simulink library "ad_blocks"  (R2017a)
settings: Solver=VariableStepAuto  StartTime=0.0  StopTime=10.0  RelTol=1e-3
undefined symbols (not defined in the file or in its folder): DiscIntNeverNeededParam
undefined symbols (not defined in the file): BatchSize, densesize, features1, features2, filtersize1
libraries: ad_blocks x23, simulink x5, dspindex x2
(part 1 of 2)
settings Model: Creator=percro2  LastModifiedBy=eruffaldi

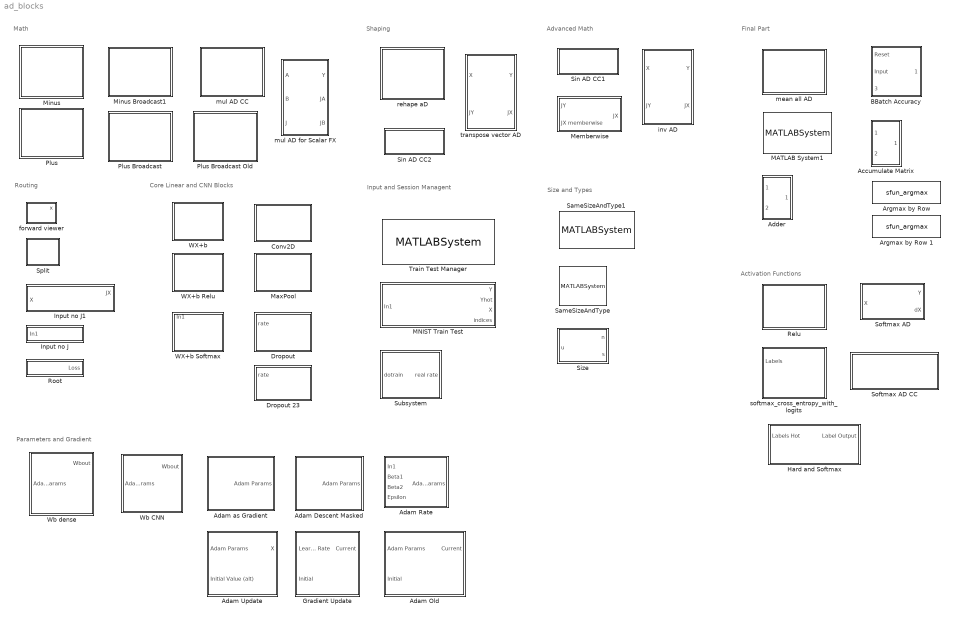
== system ad_blocks ==
  note: Advanced Math
  note: Shaping
  note: Math
  note: Size and Types
  note: Input and Session Managent
  note: Final Part
  note: Activation Functions
  note: Parameters and Gradient
  note: Routing
  note: Core Linear and CNN Blocks
  Accumulate Matrix : Subsystem  mask{Inputs=2}
      mask Callback Inputs:
      | x = gcb;
      | s = gcb;
      | asked = max(1,str2num(get_param(gcb,'Inputs')));
      | 
      | bcon = [x '/Matrix Concatenate'];
      | actual = str2num(get_param(bcon,'NumInputs'));
      | 
      | if asked == actual
      | else
      | bconL = bcon(length(x)+2:end);
      | 
      | if asked > actual
      |     set_param(bcon,'NumInputs',num2str(asked));
      |     bin1 = ([x '/In1']);
      |     bsh1 = ([x '/Reshape1']);
      |     bin1L = bin1(length(x)+2:end);
      |     bsh1L = bsh1(length(x)+2:end);
      |     for I=actual+1:asked
      |         bin = sprintf([x '/In%d'],I);
      |         bsh = sprintf([x '/Reshape%d'],I);
      |         binL = bin(length(x)+2:end);
      |         bshL = bsh(length(x)+2:end);
      |         % clone In and Reshape
      |         add_block(bin1,bin);
      |         add_block(bsh1,bsh);
      |         add_line(s,[binL '/1'],[bshL '/1']);
      |         add_line(s,[bshL '/1'],[bconL sprintf('/%d',I)]);
      |     end
      | else
      |     % remove
      |     for I=actual:-1:asked+1
      |         bin = sprintf([x '/In%d'],I);
      |         bsh = sprintf([x '/Reshape%d'],I);
      |         binL = bin(length(x)+2:end);
      |         bshL = bsh(length(x)+2:end);
      | 
      |         try
      |         delete_line(s,[binL '/1'],[bshL '/1']);
      |         catch me
      |         end
      |         try
      |         delete_line(s,[bshL '/1'],[bconL sprintf('/%d',I)]);
      |         catch me
      |         end
      |         try
      |         delete_block(bin);
      |         catch me
      |         end
      |         try
      |         delete_block(bsh);
      |         catch me
      |         end
      |     end
      |     set_param(bcon,'NumInputs',num2str(asked));
      | end
      | end
  Adam Descent Masked : Subsystem  mask{learningrate=1e-4, beta1=0.9, beta2=0.9999, epsilon=1e-8, adam=on}
      mask prompts: learningrate "Learning Rate"; adam "Check for Adam"
  Adam Old : Subsystem
  Adam Rate : Subsystem
  Adam Update : Subsystem
  Adam as Gradient : Subsystem  mask{learningrate=0.5}
  Adder : Subsystem
  "Argmax by Row " : M-S-Function  FunctionName=sfun_argmax
  Argmax by Row 1 : M-S-Function  FunctionName=sfun_argmax
  BBatch Accuracy : Subsystem
  Conv2D : Subsystem  mask{stride=[1,2,2,1], padding=-1}
      mask prompts: padding "padding (-1 auto)"
  Dropout : Subsystem
  Dropout 23 : Subsystem
  Gradient Update : Subsystem
  Hard and Softmax : Subsystem
  Input no J : Subsystem
      mask Display: disp('Input Only');
  Input no J1 : Subsystem
      mask Display: disp('Input and Gradient Only');
  MATLAB System1 : MATLABSystem  System=ArgmaxSystemD2  SimulateUsing=Code generation
      mask Type: ArgmaxSystemD2
      mask Display:
      | disp('ArgmaxSystemD2');
      | port_label('input',1,'x');
      | port_label('output',1,'y');
  MNIST Train Test : Subsystem
  MaxPool : Subsystem  mask{stride=[1,2,2,1], ksize=[1,2,2,1], padding=-1}
      mask prompts: padding "padding (-1 means auto)"
  Memberwise : Subsystem
  "Minus " : Subsystem
  Minus Broadcast1 : Subsystem
  Plus : Subsystem
  Plus Broadcast : Subsystem
  Plus Broadcast Old : Subsystem
  Relu : Subsystem
  Root : Subsystem  Description=Top level AD block: gets the incoming value, pushes the scalar 1 gradient
      mask Display: disp('Gradient Root');
  SameSizeAndType : MATLABSystem
  SameSizeAndType1 : MATLABSystem  System=samesizetype_sys  SimulateUsing=Code generation
      mask Type: samesizetype_sys
      mask Display:
      | disp('samesizetype_sys');
      | port_label('input',1,'uref');
      | port_label('input',2,'u');
      | port_label('output',1,'y');
  Sin AD CC1 : Subsystem
      mask Display: disp('inv(x)');
  Sin AD CC2 : Subsystem
      mask Display: disp('transpose(x)');
  Size : MATLAB Function  TreatAsAtomicUnit=on
  Softmax AD : Subsystem
      mask Display: image('softmax.png');
  Softmax AD CC : Subsystem
      mask Display: image('softmax.png');
  Split : Subsystem
  Subsystem : Subsystem  mask{dropout_rate=0.2}
      mask prompts: dropout_rate "Dropout Rate"
  Train Test Manager : MATLABSystem  System=train_test_mgr  testsize=10000  trainsize=60000  skiptrain=0  epochs=2  batchsize=BatchSize  SimulateUsing=Interpreted execution
      mask Type: train_test_mgr
      mask Display:
      | disp('train_test_mgr');
      | port_label('output',1,'dotrain');
      | port_label('output',2,'instop');
      | port_label('output',3,'samples');
      | port_label('output',4,'iteration');
      | port_label('output',5,'newepoch');
  "WX+b " : Subsystem
  WX+b Relu : Subsystem
  WX+b Softmax : Subsystem
  Wb CNN : Subsystem  mask{K=filtersize1, Fi=1, Fo=features1}
      mask prompts: K "Filter Size"; Fi "In Features"; Fo "Out Features"
  Wb dense : Subsystem  mask{wshape=[7*7*features2,densesize]}
      mask prompts: wshape "W Shape"
  forward viewer : Subsystem
  inv AD : Subsystem
  mean all AD : Subsystem
  mul AD CC : Subsystem
  mul AD for Scalar FX : Subsystem
  rehape aD : Subsystem  mask{shape=[-1,28,28,1]}
      mask prompts: shape "New Shape"
  softmax_cross_entropy_with_logits : Subsystem
  transpose vector AD : Subsystem

== system ad_blocks/Accumulate Matrix ==
  In1 : Inport
  In2 : Inport  Port=2
  Matrix Concatenate : Concatenate  Mode=Multidimensional array  ConcatenateDimension=2
  Reshape1 : Reshape
  Reshape2 : Reshape
  ReshapeX : Reshape  OutputDimensionality=Derive from reference input port
  Sum of Elements : Sum  Inputs=+  CollapseMode=Specified dimension  CollapseDim=2
  Out1 : Outport
  wires:
  Reshape2/1 -> Matrix Concatenate/2
  In2/1 -> Reshape2/1
  ReshapeX/1 -> Out1/1
  Matrix Concatenate/1 -> Sum of Elements/1
  Reshape1/1 -> Matrix Concatenate/1
  In1/1 -> ReshapeX/2, Reshape1/1
  Sum of Elements/1 -> ReshapeX/1

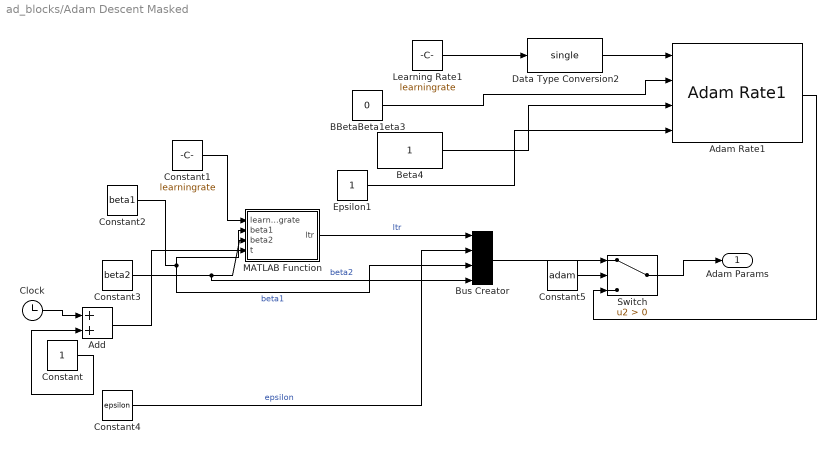
== system ad_blocks/Adam Descent Masked ==
  Adam Rate1 : ad_blocks/Adam as Gradient/Adam Rate1
  Add : Sum
  BBetaBeta1eta3 : Constant  Value=0  OutDataTypeStr=Inherit: Inherit via back propagation
  Beta4 : Constant  OutDataTypeStr=Inherit: Inherit via back propagation
  Bus Creator : BusCreator  Inputs=4
  Clock : Clock
  Constant : Constant
  Constant1 : Constant  Value=learningrate  OutDataTypeStr=Inherit: Inherit via back propagation
  Constant2 : Constant  Value=beta1  OutDataTypeStr=Inherit: Inherit via back propagation
  Constant3 : Constant  Value=beta2  OutDataTypeStr=Inherit: Inherit via back propagation
  Constant4 : Constant  Value=epsilon  OutDataTypeStr=Inherit: Inherit via back propagation
  Constant5 : Constant  Value=adam
  Data Type Conversion2 : DataTypeConversion  OutDataTypeStr=single
  Epsilon1 : Constant  OutDataTypeStr=Inherit: Inherit via back propagation
  Learning Rate1 : Constant  Value=learningrate
  MATLAB Function : MATLAB Function  TreatAsAtomicUnit=on
  Switch : Switch  Criteria=u2 > Threshold
  Adam Params : Outport
  wires:
  Constant1/1 -> MATLAB Function/1(learningrate)
  Constant2/1 -> Bus Creator/3, MATLAB Function/2(beta1)  "beta1"
  Constant3/1 -> Bus Creator/4, MATLAB Function/3(beta2)  "beta2"
  Constant4/1 -> Bus Creator/2  "epsilon"
  MATLAB Function/1(ltr) -> Bus Creator/1  "ltr"
  Constant/1 -> Add/2
  Clock/1 -> Add/1
  Add/1 -> MATLAB Function/4(t)
  Beta4/1 -> Adam Rate1/3
  BBetaBeta1eta3/1 -> Adam Rate1/2
  Epsilon1/1 -> Adam Rate1/4
  Learning Rate1/1 -> Data Type Conversion2/1
  Data Type Conversion2/1 -> Adam Rate1/1
  Bus Creator/1 -> Switch/1
  Adam Rate1/1 -> Switch/3
  Switch/1 -> Adam Params/1
  Constant5/1 -> Switch/2

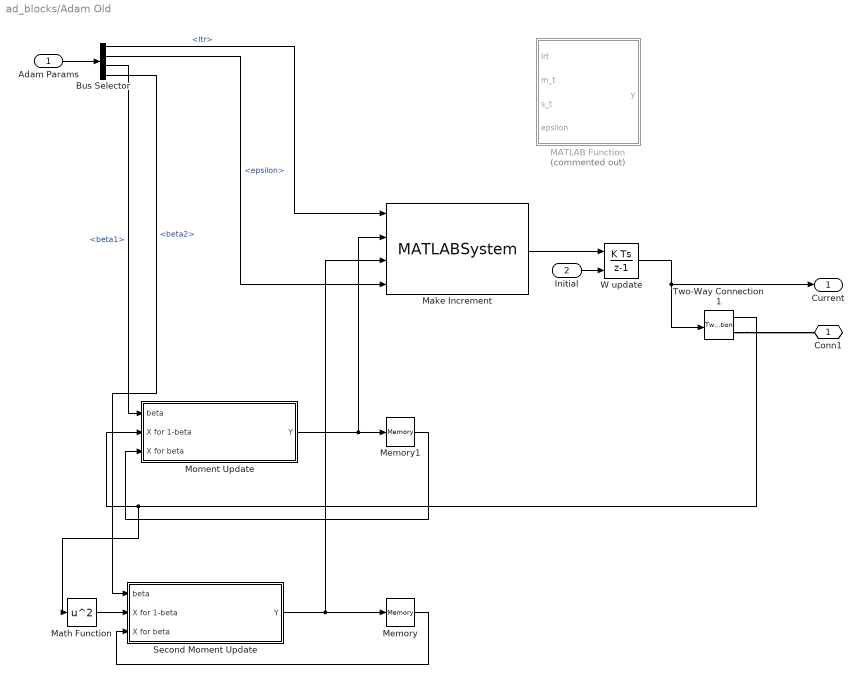
== system ad_blocks/Adam Old ==
  Adam Params : Inport
  Initial : Inport  Port=2
  Bus Selector : BusSelector  OutputSignals=ltr,epsilon,beta1,beta2
  MATLAB Function : MATLAB Function  Commented=on  TreatAsAtomicUnit=on
  Make Increment : MATLABSystem  System=adam_updateSystem  SimulateUsing=Code generation
      mask Type: adam_updateSystem
      mask Display:
      | disp('adam_updateSystem');
      | port_label('input',1,'lrt');
      | port_label('input',2,'m_t');
      | port_label('input',3,'s_t');
      | port_label('input',4,'epsilon');
      | port_label('output',1,'y');
  Math Function : Math  Operator=square  SaturateOnIntegerOverflow=on
  Memory : Memory
  Memory1 : Memory
  Moment Update : Subsystem
  Second Moment Update : Subsystem
  Two-Way Connection1 : TwoWayConnection
  W update : DiscreteIntegrator  InitialConditionSource=external  InitialConditionSetting=State (most efficient)  SampleTime=-1  ICPrevOutput=DiscIntNeverNeededParam  ICPrevScaledInput=DiscIntNeverNeededParam
  Conn1 : PMIOPort  Port=1  Side=Right
  Current : Outport
  wires:
  Make Increment/1 -> W update/1
  Bus Selector/2 -> Make Increment/4  "<epsilon>"
  Moment Update/1(Y) -> Make Increment/2, Memory1/1
  Second Moment Update/1(Y) -> Make Increment/3, Memory/1
  Math Function/1 -> Second Moment Update/2(X for 1-beta)
  Two-Way Connection1/1 -> Moment Update/2(X for 1-beta), Math Function/1
  Memory/1 -> Second Moment Update/3(X for beta)
  Bus Selector/4 -> Second Moment Update/1(beta)  "<beta2>"
  Bus Selector/3 -> Moment Update/1(beta)  "<beta1>"
  Memory1/1 -> Moment Update/3(X for beta)
  Bus Selector/1 -> Make Increment/1  "<ltr>"
  Adam Params/1 -> Bus Selector/1
  W update/1 -> Current/1, Two-Way Connection1/1
  Initial/1 -> W update/2
  connections:
  Two-Way Connection1/RConn1 -- Conn1/RConn1

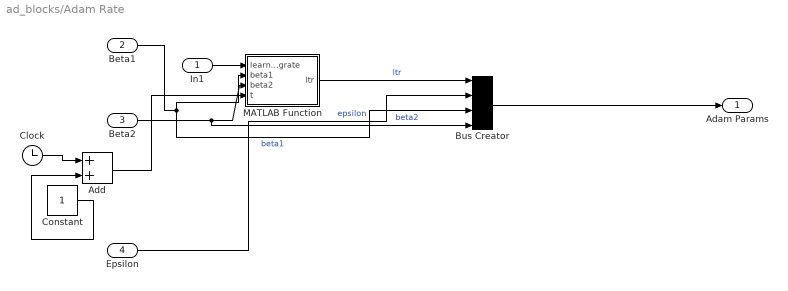
== system ad_blocks/Adam Rate ==
  In1 : Inport
  Beta1 : Inport  Port=2
  Beta2 : Inport  Port=3
  Epsilon : Inport  Port=4
  Add : Sum
  Bus Creator : BusCreator  Inputs=4
  Clock : Clock
  Constant : Constant
  MATLAB Function : MATLAB Function  TreatAsAtomicUnit=on
  Adam Params : Outport
  wires:
  In1/1 -> MATLAB Function/1(learningrate)
  Beta1/1 -> Bus Creator/3, MATLAB Function/2(beta1)  "beta1"
  Beta2/1 -> Bus Creator/4, MATLAB Function/3(beta2)  "beta2"
  Epsilon/1 -> Bus Creator/2  "epsilon"
  MATLAB Function/1(ltr) -> Bus Creator/1  "ltr"
  Bus Creator/1 -> Adam Params/1
  Constant/1 -> Add/2
  Clock/1 -> Add/1
  Add/1 -> MATLAB Function/4(t)

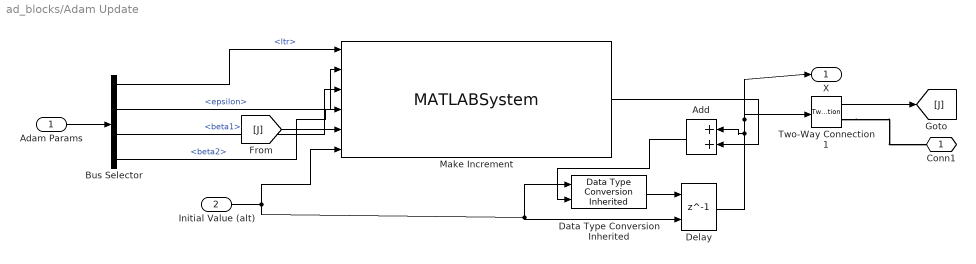
== system ad_blocks/Adam Update ==
  Adam Params : Inport
  Initial Value (alt) : Inport  Port=2
  Add : Sum  OutDataTypeStr=Inherit: Same as first input
  Bus Selector : BusSelector  OutputSignals=ltr,epsilon,beta1,beta2
  Data Type Conversion Inherited : simulink/Signal Attributes/Data Type Conversion Inherited  ConvertRealWorld=Real World Value  DoSatur=off
      settings: SourceProductName=Simulink  SourceProductBaseCode=SL
  Delay : Delay  DelayLength=1  InitialConditionSource=Input port
      settings: InputPortMap=u0,p4
  Make Increment : MATLABSystem  System=adam_updateSystem  SimulateUsing=Interpreted execution
      mask Type: adam_updateSystem
      mask Display:
      | disp('adam_updateSystem');
      | port_label('input',1,'learning_rate');
      | port_label('input',2,'epsilon');
      | port_label('input',3,'beta1');
      | port_label('input',4,'beta2');
      | port_label('input',5,'gradient');
      | port_label('input',6,'initial_for_size');
      | port_label('output',1,'effective_gradient');
  Two-Way Connection1 : TwoWayConnection
  Conn1 : PMIOPort  Port=1  Side=Right
  X : Outport
  wires:
  Adam Params/1 -> Bus Selector/1
  Bus Selector/1 -> Make Increment/1  "<ltr>"
  Bus Selector/2 -> Make Increment/2  "<epsilon>"
  Bus Selector/3 -> Make Increment/3  "<beta1>"
  Bus Selector/4 -> Make Increment/4  "<beta2>"
  Initial Value (alt)/1 -> Data Type Conversion Inherited/1, Delay/2, Make Increment/6
  Delay/1 -> Add/1, X/1, Two-Way Connection1/1
  [J] -> Make Increment/5
  Two-Way Connection1/1 -> [J]
  Make Increment/1 -> Add/2
  Data Type Conversion Inherited/1 -> Delay/1
  Add/1 -> Data Type Conversion Inherited/2
  connections:
  Two-Way Connection1/RConn1 -- Conn1/RConn1

== system ad_blocks/Adam as Gradient ==
  Adam Rate1 : Subsystem
  BBetaBeta1eta3 : Constant  Value=0  OutDataTypeStr=Inherit: Inherit via back propagation
  Beta4 : Constant  OutDataTypeStr=Inherit: Inherit via back propagation
  Data Type Conversion2 : DataTypeConversion  OutDataTypeStr=single
  Epsilon1 : Constant  OutDataTypeStr=Inherit: Inherit via back propagation
  Learning Rate1 : Constant  Value=learningrate
  Adam Params : Outport
  wires:
  Data Type Conversion2/1 -> Adam Rate1/1(In1)
  Adam Rate1/1(Adam Params) -> Adam Params/1
  Epsilon1/1 -> Adam Rate1/4(Epsilon)
  BBetaBeta1eta3/1 -> Adam Rate1/2(Beta1)
  Beta4/1 -> Adam Rate1/3(Beta2)
  Learning Rate1/1 -> Data Type Conversion2/1

== system ad_blocks/Adder ==
  Initial : Inport
  Input : Inport  Port=2
  Add : Sum
  Delay : Delay  DelayLength=1  InitialConditionSource=Input port
      settings: InputPortMap=u0,p4
  Output : Outport
  wires:
  Delay/1 -> Add/1
  Add/1 -> Output/1, Delay/1
  Initial/1 -> Delay/2
  Input/1 -> Add/2

== system ad_blocks/BBatch Accuracy ==
  Reset : Inport
  Input : Inport  Port=2
  Total Count : Inport  Port=3
  Data Type Conversion1 : DataTypeConversion
  Divide : Product  Inputs=*/
  Sum of Elements : Sum  Inputs=+
  W update : DiscreteIntegrator  ExternalReset=rising  InitialConditionSetting=State (most efficient)  SampleTime=-1  ICPrevOutput=DiscIntNeverNeededParam  ICPrevScaledInput=DiscIntNeverNeededParam
  Accuracy : Outport
  wires:
  Input/1 -> Sum of Elements/1
  W update/1 -> Divide/1
  Total Count/1 -> Divide/2
  Divide/1 -> Accuracy/1
  Sum of Elements/1 -> Data Type Conversion1/1
  Data Type Conversion1/1 -> W update/1
  Reset/1 -> W update/2

== system ad_blocks/Conv2D ==
  Gradient : MATLABSystem  System=conv2d_grad  SimulateUsing=Interpreted execution
      mask Type: conv2d_grad
      mask Display:
      | disp('conv2d_grad');
      | port_label('input',1,'U_B_Ph_Pw_Q');
      | port_label('input',2,'A_B_I_C');
      | port_label('input',3,'W_K_C_Q');
      | port_label('input',4,'Sel_PKC_IC');
      | port_label('input',5,'Xp_BP_KC');
      | port_label('output',1,'dzdx_B_Ph_Pw_Q');
      | port_label('output',2,'dzdW_K_C_Q');
  Setup : MATLABSystem  System=conv2d_setup  padding=padding  stride=stride  SimulateUsing=Interpreted execution
      mask Type: conv2d_setup
      mask Display:
      | disp('conv2d_setup');
      | port_label('input',1,'X');
      | port_label('input',2,'W');
      | port_label('output',1,'Sel_PKC_IC');
      | port_label('output',2,'Zero_Ph_Pw');
  Two-Way Connection1 : TwoWayConnection
  Two-Way Connection2 : TwoWayConnection
  Two-Way Connection3 : TwoWayConnection
  Value : MATLABSystem  System=conv2d_eval  padding=-1  stride=stride  SimulateUsing=Interpreted execution
      mask Type: conv2d_eval
      mask Display:
      | disp('conv2d_eval');
      | port_label('input',1,'A_B_I_C');
      | port_label('input',2,'W_K_C_Q');
      | port_label('input',3,'Sel_PKC_IC');
      | port_label('input',4,'Zero_Ph_PW');
      | port_label('output',1,'y_B_Ph_Pw_Q');
      | port_label('output',2,'Xp_BP_KC');
  X : PMIOPort  Port=1  Side=Left
  W : PMIOPort  Port=2  Side=Left
  Y : PMIOPort  Port=3  Side=Right
  wires:
  Two-Way Connection1/1 -> Gradient/2, Value/1, Setup/1
  Value/1 -> Two-Way Connection2/1
  Two-Way Connection3/1 -> Gradient/3, Value/2, Setup/2
  Gradient/1 -> Two-Way Connection1/1
  Gradient/2 -> Two-Way Connection3/1
  Two-Way Connection2/1 -> Gradient/1
  Value/2 -> Gradient/5
  Setup/1 -> Gradient/4, Value/3
  Setup/2 -> Value/4
  connections:
  X/RConn1 -- Two-Way Connection1/RConn1
  Two-Way Connection2/RConn1 -- Y/RConn1
  W/RConn1 -- Two-Way Connection3/RConn1

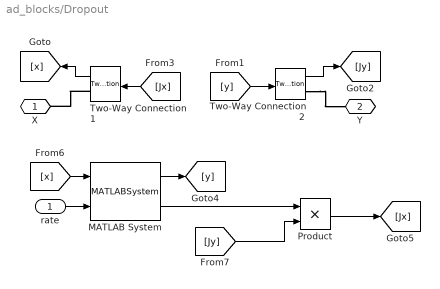
== system ad_blocks/Dropout ==
  rate : Inport
  MATLAB System : MATLABSystem  System=dropout_sys  SimulateUsing=Code generation
      mask Type: dropout_sys
      mask Display:
      | disp('dropout_sys');
      | port_label('input',1,'x');
      | port_label('input',2,'rate');
      | port_label('output',1,'y');
      | port_label('output',2,'mask');
  Product : Product
  Two-Way Connection1 : TwoWayConnection
  Two-Way Connection2 : TwoWayConnection
  X : PMIOPort  Port=1  Side=Left
  Y : PMIOPort  Port=2  Side=Right
  wires:
  rate/1 -> MATLAB System/2
  [Jx] -> Two-Way Connection1/1
  [y] -> Two-Way Connection2/1
  Two-Way Connection2/1 -> [Jy]
  Two-Way Connection1/1 -> [x]
  [x] -> MATLAB System/1
  MATLAB System/1 -> [y]
  Product/1 -> [Jx]
  MATLAB System/2 -> Product/1
  [Jy] -> Product/2
  connections:
  Two-Way Connection2/RConn1 -- Y/RConn1
  Two-Way Connection1/RConn1 -- X/RConn1

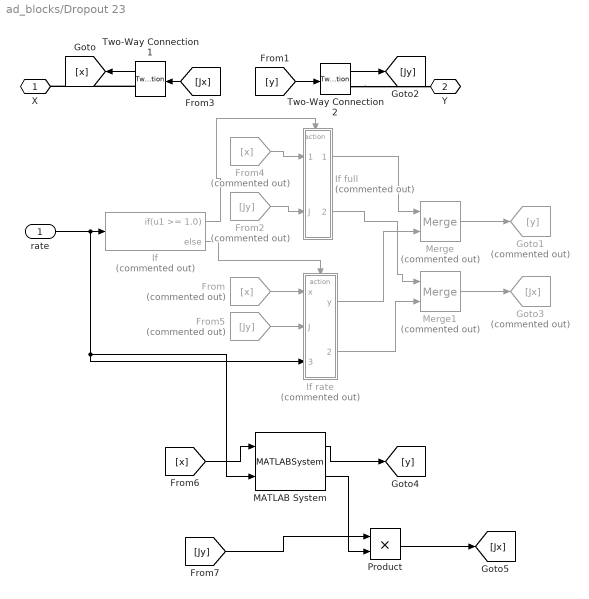
== system ad_blocks/Dropout 23 ==
  rate : Inport
  From : From  Commented=on  GotoTag=x
  From2 : From  Commented=on  GotoTag=Jy
  From4 : From  Commented=on  GotoTag=x
  From5 : From  Commented=on  GotoTag=Jy
  Goto1 : Goto  Commented=on  GotoTag=y
  Goto3 : Goto  Commented=on  GotoTag=Jx
  If : If  Commented=on  IfExpression=u1 >= 1.0
  If full : Subsystem  Commented=on  TreatAsAtomicUnit=on
  If rate : Subsystem  Commented=on  TreatAsAtomicUnit=on
  MATLAB System : MATLABSystem  System=dropout23_sys  SimulateUsing=Code generation
      mask Type: dropout23_sys
      mask Display:
      | disp('dropout23_sys');
      | port_label('input',1,'x');
      | port_label('input',2,'rate');
      | port_label('output',1,'y');
      | port_label('output',2,'mask');
  Merge : Merge  Commented=on
  Merge1 : Merge  Commented=on
  Product : Product
  Two-Way Connection1 : TwoWayConnection
  Two-Way Connection2 : TwoWayConnection
  X : PMIOPort  Port=1  Side=Left
  Y : PMIOPort  Port=2  Side=Right
  wires:
  rate/1 -> MATLAB System/2, If rate/3(rate), If/1
  If/1 -> If full/Action
  If/2 -> If rate/Action
  If full/1(y) -> Merge/1
  If rate/1(y) -> Merge/2
  If full/2(Jx) -> Merge1/1
  If rate/2(Jx) -> Merge1/2
  Merge/1 -> Goto1/1
  Merge1/1 -> Goto3/1
  [Jx] -> Two-Way Connection1/1
  [y] -> Two-Way Connection2/1
  Two-Way Connection2/1 -> [Jy]
  Two-Way Connection1/1 -> [x]
  From/1 -> If rate/1(x)
  From2/1 -> If full/2(J)
  From4/1 -> If full/1(x)
  From5/1 -> If rate/2(J)
  [x] -> MATLAB System/1
  MATLAB System/1 -> [y]
  Product/1 -> [Jx]
  MATLAB System/2 -> Product/2
  [Jy] -> Product/1
  connections:
  Two-Way Connection2/RConn1 -- Y/RConn1
  Two-Way Connection1/RConn1 -- X/RConn1

== system ad_blocks/Gradient Update ==
  Learning Rate : Inport
  Initial : Inport  Port=2
  Adder : ad_blocks/Adder
  Product : Product
  Two-Way Connection1 : TwoWayConnection
  Unary Minus : UnaryMinus
  Conn1 : PMIOPort  Port=1  Side=Right
  Current : Outport
  wires:
  Learning Rate/1 -> Unary Minus/1
  Two-Way Connection1/1 -> Product/1
  Adder/1 -> Current/1, Two-Way Connection1/1
  Unary Minus/1 -> Product/2
  Initial/1 -> Adder/1
  Product/1 -> Adder/2
  connections:
  Two-Way Connection1/RConn1 -- Conn1/RConn1

== system ad_blocks/Hard and Softmax ==
  Labels Hot : Inport
  MATLAB System1 : ad_blocks/MATLAB System1  SimulateUsing=Code generation
  forward viewer2 : ad_blocks/forward viewer  SystemSampleTime=-1
  softmax_cross_entropy_with_logits : ad_blocks/softmax_cross_entropy_with_logits
  X : PMIOPort  Port=1  Side=Left
  Y : PMIOPort  Port=2  Side=Right
  Label Output : Outport
  wires:
  forward viewer2/1 -> MATLAB System1/1
  Labels Hot/1 -> softmax_cross_entropy_with_logits/1
  MATLAB System1/1 -> Label Output/1
  connections:
  softmax_cross_entropy_with_logits/RConn1 -- Y/RConn1
  forward viewer2/RConn1 -- softmax_cross_entropy_with_logits/LConn1
  X/RConn1 -- forward viewer2/LConn1

== system ad_blocks/Input no J ==
  In1 : Inport
  Terminator : Terminator
  Two-Way Connection1 : TwoWayConnection
  Conn1 : PMIOPort  Port=1  Side=Right
  wires:
  In1/1 -> Two-Way Connection1/1
  Two-Way Connection1/1 -> Terminator/1
  connections:
  Conn1/RConn1 -- Two-Way Connection1/RConn1

== system ad_blocks/Input no J1 ==
  X : Inport
  Two-Way Connection1 : TwoWayConnection
  (X,JX) : PMIOPort  Port=1  Side=Right
  JX : Outport
  wires:
  Two-Way Connection1/1 -> JX/1
  X/1 -> Two-Way Connection1/1
  connections:
  (X,JX)/RConn1 -- Two-Way Connection1/RConn1

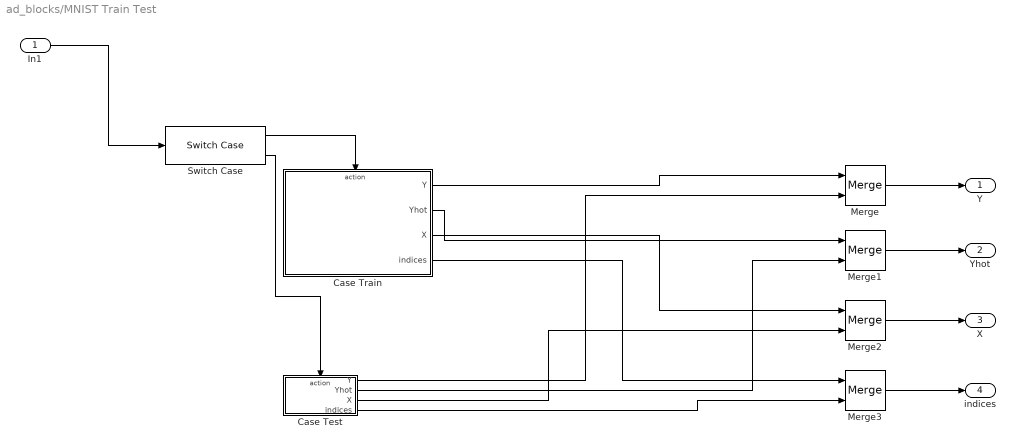
== system ad_blocks/MNIST Train Test ==
  In1 : Inport
  Case Test : Subsystem  TreatAsAtomicUnit=on
  Case Train : Subsystem  TreatAsAtomicUnit=on
  Merge{,1..3} (4 alike) : Merge
  Switch Case : SwitchCase
  "Y " : Outport
  Yhot : Outport  Port=2
  X : Outport  Port=3
  indices : Outport  Port=4
  wires:
  In1/1 -> Switch Case/1
  Switch Case/1 -> Case Train/Action
  Switch Case/2 -> Case Test/Action
  Case Train/1(Y) -> Merge/1
  Case Train/2(Yhot) -> Merge1/1
  Case Train/3(X) -> Merge2/1
  Case Test/1(Y) -> Merge/2
  Case Test/2(Yhot) -> Merge1/2
  Case Test/3(X) -> Merge2/2
  Merge/1 -> "Y "/1
  Merge1/1 -> Yhot/1
  Merge2/1 -> X/1
  Merge3/1 -> indices/1
  Case Test/4(indices) -> Merge3/2
  Case Train/4(indices) -> Merge3/1

== system ad_blocks/MaxPool ==
  note: setup is based on the constant size extraction, then it produces in a constant way the indices
      | then the evaluation produces also the indices I that are finally used in the gradient
  Gradient : MATLABSystem  System=maxpool_grad  ksize=ksize  strides=stride  SimulateUsing=Interpreted execution
      mask Type: maxpool_grad
      mask Display:
      | disp('maxpool_grad');
      | port_label('input',1,'U_B_Ph_Pw_Q');
      | port_label('input',2,'argmaxbase');
      | port_label('input',3,'maxindices_BPC');
      | port_label('input',4,'argmaxbasescale');
      | port_label('input',5,'Zero_Ph_Pw');
      | port_label('input',6,'X_B_I_C');
      | port_label('input',7,'Sel_PCK_IC');
      | port_label('input',8,'Sel_PCK_IC_A');
      | port_label('output',1,'J_BIC');
  Setup : MATLABSystem  System=maxpool_setup  ksize=ksize  strides=stride  padding=padding  SimulateUsing=Interpreted execution
      mask Type: maxpool_setup
      mask Display:
      | disp('maxpool_setup');
      | port_label('input',1,'X');
      | port_label('output',1,'Sel_PCK_IC');
      | port_label('output',2,'argmaxbase');
      | port_label('output',3,'argmaxbasescale');
      | port_label('output',4,'Zero_Ph_Pw');
      | port_label('output',5,'Sel_PCK_IC_A');
  Two-Way Connection1 : TwoWayConnection
  Two-Way Connection2 : TwoWayConnection
  "Value " : MATLABSystem  System=maxpool_eval  strides=stride  ksize=ksize  SimulateUsing=Interpreted execution
      mask Type: maxpool_eval
      mask Display:
      | disp('maxpool_eval');
      | port_label('input',1,'X_B_I_C');
      | port_label('input',2,'Sel_PCK_IC');
      | port_label('input',3,'Zero_Ph_Pw');
      | port_label('output',1,'y_B_P_C');
      | port_label('output',2,'maxindices_BPC');
  X : PMIOPort  Port=1  Side=Left
  Y : PMIOPort  Port=2  Side=Right
  wires:
  Two-Way Connection1/1 -> Setup/1, Gradient/6, "Value "/1
  Gradient/1 -> Two-Way Connection1/1
  "Value "/1 -> Two-Way Connection2/1
  Setup/1 -> Gradient/7, "Value "/2
  Two-Way Connection2/1 -> Gradient/1
  Setup/2 -> Gradient/2
  Setup/4 -> "Value "/3, Gradient/5
  Setup/3 -> Gradient/4
  "Value "/2 -> Gradient/3
  Setup/5 -> Gradient/8
  connections:
  Y/RConn1 -- Two-Way Connection2/RConn1
  X/RConn1 -- Two-Way Connection1/RConn1

== system ad_blocks/Memberwise ==
  JY : Inport
  JX memberwise : Inport  Port=2
  Product : Product
  JX : Outport
  wires:
  JY/1 -> Product/1
  JX memberwise/1 -> Product/2
  Product/1 -> JX/1

== system ad_blocks/Minus  ==
  Add : Sum  Inputs=+-
  Gain : Gain  Gain=-1
  Two-Way Connection1 : TwoWayConnection
  Two-Way Connection2 : TwoWayConnection
  Two-Way Connection4 : TwoWayConnection
  A : PMIOPort  Port=1  Side=Left
  B : PMIOPort  Port=2  Side=Left
  Y : PMIOPort  Port=3  Side=Right
  wires:
  Two-Way Connection2/1 -> Add/1
  Two-Way Connection1/1 -> Gain/1, Two-Way Connection2/1
  Add/1 -> Two-Way Connection1/1
  Gain/1 -> Two-Way Connection4/1
  Two-Way Connection4/1 -> Add/2
  connections:
  Y/RConn1 -- Two-Way Connection1/RConn1
  Two-Way Connection4/RConn1 -- B/RConn1
  A/RConn1 -- Two-Way Connection2/RConn1

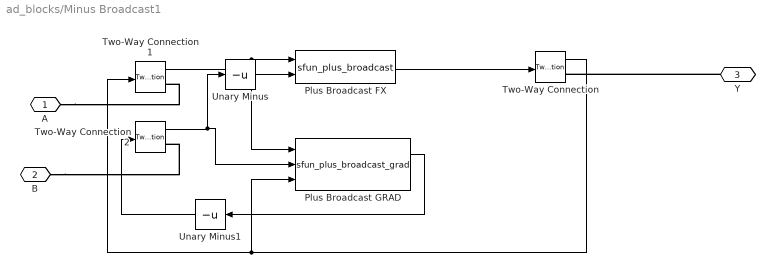
== system ad_blocks/Minus Broadcast1 ==
  Plus Broadcast FX : M-S-Function  FunctionName=sfun_plus_broadcast
  Plus Broadcast GRAD : M-S-Function  FunctionName=sfun_plus_broadcast_grad
  Two-Way Connection : TwoWayConnection
  Two-Way Connection1 : TwoWayConnection
  Two-Way Connection2 : TwoWayConnection
  Unary Minus : UnaryMinus
  Unary Minus1 : UnaryMinus
  A : PMIOPort  Port=1  Side=Left
  B : PMIOPort  Port=2  Side=Left
  Y : PMIOPort  Port=3  Side=Right
  wires:
  Two-Way Connection/1 -> Plus Broadcast GRAD/3, Two-Way Connection1/1
  Plus Broadcast GRAD/1 -> Unary Minus1/1
  Two-Way Connection2/1 -> Unary Minus/1, Plus Broadcast GRAD/2
  Two-Way Connection1/1 -> Plus Broadcast FX/1, Plus Broadcast GRAD/1
  Plus Broadcast FX/1 -> Two-Way Connection/1
  Unary Minus/1 -> Plus Broadcast FX/2
  Unary Minus1/1 -> Two-Way Connection2/1
  connections:
  B/RConn1 -- Two-Way Connection2/RConn1
  A/RConn1 -- Two-Way Connection1/RConn1
  Y/RConn1 -- Two-Way Connection/RConn1

== system ad_blocks/Plus ==
  Add : Sum
  Two-Way Connection : TwoWayConnection
  Two-Way Connection1 : TwoWayConnection
  Two-Way Connection2 : TwoWayConnection
  A : PMIOPort  Port=1  Side=Left
  B : PMIOPort  Port=2  Side=Left
  Y : PMIOPort  Port=3  Side=Right
  wires:
  Two-Way Connection2/1 -> Add/2
  Two-Way Connection1/1 -> Add/1
  Two-Way Connection/1 -> Two-Way Connection2/1, Two-Way Connection1/1
  Add/1 -> Two-Way Connection/1
  connections:
  B/RConn1 -- Two-Way Connection2/RConn1
  A/RConn1 -- Two-Way Connection1/RConn1
  Y/RConn1 -- Two-Way Connection/RConn1

== system ad_blocks/Plus Broadcast ==
  Two-Way Connection : TwoWayConnection
  Two-Way Connection1 : TwoWayConnection
  Two-Way Connection2 : TwoWayConnection
  function : MATLABSystem  System=SumBroadcast  SimulateUsing=Code generation
      mask Type: SumBroadcast
      mask Display:
      | disp('SumBroadcast');
      | port_label('input',1,'ul');
      | port_label('input',2,'ur');
      | port_label('output',1,'y');
  gradient : MATLABSystem  System=SumBroadcastGrad  SimulateUsing=Code generation
      mask Type: SumBroadcastGrad
      mask Display:
      | disp('SumBroadcastGrad');
      | port_label('input',1,'ul');
      | port_label('input',2,'ur');
      | port_label('input',3,'J');
      | port_label('output',1,'Jl');
      | port_label('output',2,'Jr');
  A : PMIOPort  Port=1  Side=Left
  B : PMIOPort  Port=2  Side=Left
  Y : PMIOPort  Port=3  Side=Right
  wires:
  function/1 -> Two-Way Connection/1
  Two-Way Connection1/1 -> gradient/1, function/1
  Two-Way Connection2/1 -> function/2, gradient/2
  gradient/2 -> Two-Way Connection2/1
  Two-Way Connection/1 -> gradient/3
  gradient/1 -> Two-Way Connection1/1
  connections:
  Y/RConn1 -- Two-Way Connection/RConn1
  A/RConn1 -- Two-Way Connection1/RConn1
  B/RConn1 -- Two-Way Connection2/RConn1

== system ad_blocks/Plus Broadcast Old ==
  Plus Broadcast FX : M-S-Function  FunctionName=sfun_plus_broadcast
  Plus Broadcast GRAD : M-S-Function  FunctionName=sfun_plus_broadcast_grad
  Two-Way Connection : TwoWayConnection
  Two-Way Connection1 : TwoWayConnection
  Two-Way Connection2 : TwoWayConnection
  A : PMIOPort  Port=1  Side=Left
  B : PMIOPort  Port=2  Side=Left
  Y : PMIOPort  Port=3  Side=Right
  wires:
  Plus Broadcast FX/1 -> Two-Way Connection/1
  Two-Way Connection1/1 -> Plus Broadcast GRAD/1, Plus Broadcast FX/1
  Two-Way Connection2/1 -> Plus Broadcast GRAD/2, Plus Broadcast FX/2
  Plus Broadcast GRAD/1 -> Two-Way Connection2/1
  Two-Way Connection/1 -> Two-Way Connection1/1, Plus Broadcast GRAD/3
  connections:
  Y/RConn1 -- Two-Way Connection/RConn1
  A/RConn1 -- Two-Way Connection1/RConn1
  B/RConn1 -- Two-Way Connection2/RConn1

== system ad_blocks/Relu ==
  MATLAB System : MATLABSystem  System=ReluGradient_sys  SimulateUsing=Code generation
      mask Type: ReluGradient_sys
      mask Display:
      | disp('ReluGradient_sys');
      | port_label('input',1,'X');
      | port_label('input',2,'JY');
      | port_label('output',1,'JX');
  Two-Way Connection1 : TwoWayConnection
  Two-Way Connection2 : TwoWayConnection
  max(x,0) : MATLABSystem  System=Max0System  SimulateUsing=Code generation
      mask Type: Max0System
      mask Display:
      | disp('Max0System');
      | port_label('input',1,'x');
      | port_label('output',1,'y');
  X : PMIOPort  Port=1  Side=Left
  Y : PMIOPort  Port=2  Side=Right
  wires:
  Two-Way Connection1/1 -> MATLAB System/1, max(x,0)/1
  max(x,0)/1 -> Two-Way Connection2/1
  MATLAB System/1 -> Two-Way Connection1/1
  Two-Way Connection2/1 -> MATLAB System/2
  connections:
  X/RConn1 -- Two-Way Connection1/RConn1
  Two-Way Connection2/RConn1 -- Y/RConn1

== system ad_blocks/Root ==
  Constant1 : Constant  OutDataTypeStr=single
  Signal Specification : SignalSpecification  Dimensions=1
  Two-Way Connection1 : TwoWayConnection
  Conn1 : PMIOPort  Port=1  Side=Left
  Loss : Outport
  wires:
  Signal Specification/1 -> Loss/1
  Two-Way Connection1/1 -> Signal Specification/1
  Constant1/1 -> Two-Way Connection1/1
  connections:
  Conn1/RConn1 -- Two-Way Connection1/RConn1

== system ad_blocks/Sin AD CC1 ==
  Two-Way Connection : TwoWayConnection
  Two-Way Connection1 : TwoWayConnection
  inv AD : ad_blocks/inv AD
  X : PMIOPort  Port=1  Side=Left
  Y : PMIOPort  Port=2  Side=Right
  wires:
  inv AD/1 -> Two-Way Connection/1
  Two-Way Connection/1 -> inv AD/2
  Two-Way Connection1/1 -> inv AD/1
  inv AD/2 -> Two-Way Connection1/1
  connections:
  X/RConn1 -- Two-Way Connection1/RConn1
  Y/RConn1 -- Two-Way Connection/RConn1

== system ad_blocks/Sin AD CC2 ==
  Two-Way Connection : TwoWayConnection
  Two-Way Connection1 : TwoWayConnection
  transpose vector AD : ad_blocks/transpose vector AD
  X : PMIOPort  Port=1  Side=Left
  Y : PMIOPort  Port=2  Side=Right
  wires:
  transpose vector AD/2 -> Two-Way Connection1/1
  Two-Way Connection1/1 -> transpose vector AD/1
  Two-Way Connection/1 -> transpose vector AD/2
  transpose vector AD/1 -> Two-Way Connection/1
  connections:
  Y/RConn1 -- Two-Way Connection/RConn1
  X/RConn1 -- Two-Way Connection1/RConn1

== system ad_blocks/Softmax AD ==
  note: http://eli.thegreenplace.net/2016/the-softmax-function-and-its-derivative/
  note: https://github.com/Theano/Theano/blob/master/theano/tensor/nnet/nnet.py
  X : Inport
  MATLAB Function1 : MATLAB Function  TreatAsAtomicUnit=on
  MATLAB Function2 : MATLAB Function  TreatAsAtomicUnit=on
  Y : Outport
  dX : Outport  Port=2
  wires:
  MATLAB Function2/1(y) -> dX/1
  X/1 -> MATLAB Function1/1(u), MATLAB Function2/1(u)
  MATLAB Function1/1(y) -> Y/1

== system ad_blocks/Softmax AD CC ==
  Memberwise : ad_blocks/Memberwise
  Softmax AD : ad_blocks/Softmax AD  SystemSampleTime=-1
  Two-Way Connection : TwoWayConnection
  Two-Way Connection1 : TwoWayConnection
  X : PMIOPort  Port=1  Side=Left
  Y : PMIOPort  Port=2  Side=Right
  wires:
  Softmax AD/1 -> Two-Way Connection/1
  Two-Way Connection1/1 -> Softmax AD/1
  Two-Way Connection/1 -> Memberwise/1
  Memberwise/1 -> Two-Way Connection1/1
  Softmax AD/2 -> Memberwise/2
  connections:
  Y/RConn1 -- Two-Way Connection/RConn1
  X/RConn1 -- Two-Way Connection1/RConn1

== system ad_blocks/Split ==
  note: Alternatively use Clone Output
  Acciumulate Matrix : ad_blocks/Acciumulate Matrix  Inputs=2
  Two-Way Connection1 : TwoWayConnection
  Two-Way Connection2 : TwoWayConnection
  Two-Way Connection3 : TwoWayConnection
  X : PMIOPort  Port=1  Side=Left
  X1 : PMIOPort  Port=2  Side=Right
  X2 : PMIOPort  Port=3  Side=Right
  wires:
  Acciumulate Matrix/1 -> Two-Way Connection2/1
  Two-Way Connection1/1 -> Acciumulate Matrix/2
  Two-Way Connection3/1 -> Acciumulate Matrix/1
  Two-Way Connection2/1 -> Two-Way Connection3/1, Two-Way Connection1/1
  connections:
  Two-Way Connection3/RConn1 -- X2/RConn1
  X1/RConn1 -- Two-Way Connection1/RConn1
  Two-Way Connection2/RConn1 -- X/RConn1

== system ad_blocks/Subsystem ==
  dotrain : Inport
  Constant : Constant  Value=dropout_rate
  Constant1 : Constant  Value=1.0
  Switch : Switch  Criteria=u2 ~= 0
  real rate : Outport
  wires:
  Constant1/1 -> Switch/3
  Constant/1 -> Switch/1
  dotrain/1 -> Switch/2
  Switch/1 -> real rate/1

== system ad_blocks/WX+b  ==
  Plus Broadcast : ad_blocks/Plus Broadcast
  mul AD CC : ad_blocks/mul AD CC
  X : PMIOPort  Port=1  Side=Left
  W : PMIOPort  Port=2  Side=Left
  Y : PMIOPort  Port=3  Side=Right
  b : PMIOPort  Port=4  Side=Left
  connections:
  Y/RConn1 -- Plus Broadcast/RConn1
  Plus Broadcast/LConn2 -- b/RConn1
  mul AD CC/LConn1 -- X/RConn1
  mul AD CC/LConn2 -- W/RConn1
  Plus Broadcast/LConn1 -- mul AD CC/RConn1

== system ad_blocks/WX+b Relu ==
  Plus Broadcast : ad_blocks/Plus Broadcast
  Relu : ad_blocks/Relu
  mul AD CC : ad_blocks/mul AD CC
  X : PMIOPort  Port=1  Side=Left
  W : PMIOPort  Port=2  Side=Left
  Y : PMIOPort  Port=3  Side=Right
  b : PMIOPort  Port=4  Side=Left
  connections:
  Relu/RConn1 -- Y/RConn1
  Plus Broadcast/LConn2 -- b/RConn1
  mul AD CC/LConn1 -- X/RConn1
  mul AD CC/LConn2 -- W/RConn1
  Plus Broadcast/RConn1 -- Relu/LConn1
  Plus Broadcast/LConn1 -- mul AD CC/RConn1

== system ad_blocks/WX+b Softmax ==
  In1 : Inport
  Plus Broadcast : ad_blocks/Plus Broadcast
  mul AD CC : ad_blocks/mul AD CC
  softmax_cross_entropy_with_logits : ad_blocks/softmax_cross_entropy_with_logits
  X : PMIOPort  Port=1  Side=Left
  W : PMIOPort  Port=2  Side=Left
  Y : PMIOPort  Port=3  Side=Right
  b : PMIOPort  Port=4  Side=Left
  wires:
  In1/1 -> softmax_cross_entropy_with_logits/1
  connections:
  Plus Broadcast/LConn1 -- mul AD CC/RConn1
  Plus Broadcast/RConn1 -- softmax_cross_entropy_with_logits/LConn1
  mul AD CC/LConn2 -- W/RConn1
  mul AD CC/LConn1 -- X/RConn1
  Plus Broadcast/LConn2 -- b/RConn1
  softmax_cross_entropy_with_logits/RConn1 -- Y/RConn1

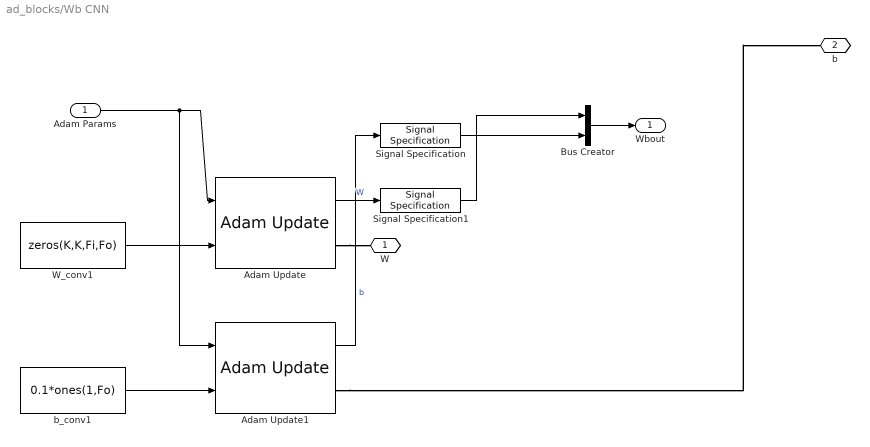
== system ad_blocks/Wb CNN ==
  Adam Params : Inport
  Adam Update : ad_blocks/Adam Update
  Adam Update1 : ad_blocks/Adam Update
  Bus Creator : BusCreator  Inputs=2
  Signal Specification : SignalSpecification  Dimensions=[Fo]
  Signal Specification1 : SignalSpecification  Dimensions=[K,K,Fi,Fo]
  W_conv1 : Constant  Value=zeros(K,K,Fi,Fo)  OutDataTypeStr=single
  b_conv1 : Constant  Value=0.1*ones(1,Fo)  OutDataTypeStr=single
  W : PMIOPort  Port=1  Side=Right
  b : PMIOPort  Port=2  Side=Right
  Wbout : Outport
  wires:
  b_conv1/1 -> Adam Update1/2
  W_conv1/1 -> Adam Update/2
  Adam Params/1 -> Adam Update/1, Adam Update1/1
  Adam Update/1 -> Signal Specification1/1  "W"
  Bus Creator/1 -> Wbout/1
  Adam Update1/1 -> Signal Specification/1  "b"
  Signal Specification/1 -> Bus Creator/2
  Signal Specification1/1 -> Bus Creator/1
  connections:
  Adam Update1/RConn1 -- b/RConn1
  Adam Update/RConn1 -- W/RConn1

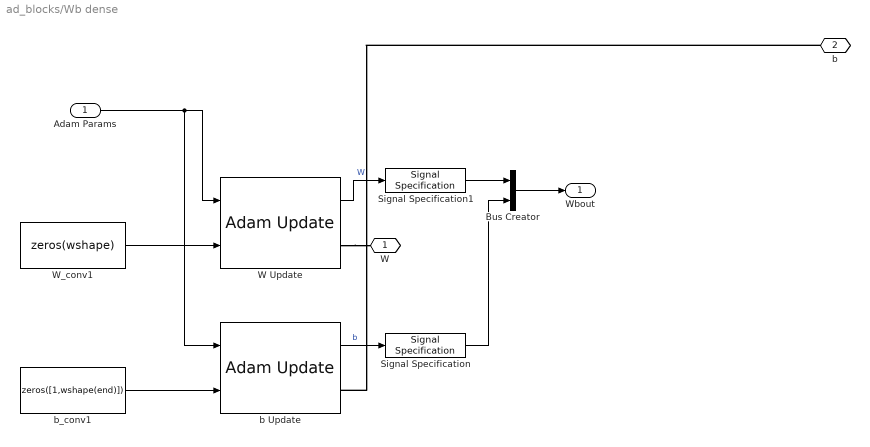
== system ad_blocks/Wb dense ==
  Adam Params : Inport
  Bus Creator : BusCreator  Inputs=2
  Signal Specification : SignalSpecification  Dimensions=[wshape(end)]
  Signal Specification1 : SignalSpecification  Dimensions=wshape
  W Update : ad_blocks/Adam Update
  W_conv1 : Constant  Value=zeros(wshape)  OutDataTypeStr=single
  b Update : ad_blocks/Adam Update
  b_conv1 : Constant  Value=zeros([1,wshape(end)])  OutDataTypeStr=single
  W : PMIOPort  Port=1  Side=Right
  b : PMIOPort  Port=2  Side=Right
  Wbout : Outport
  wires:
  b_conv1/1 -> b Update/2
  W_conv1/1 -> W Update/2
  Adam Params/1 -> b Update/1, W Update/1
  Bus Creator/1 -> Wbout/1
  W Update/1 -> Signal Specification1/1  "W"
  b Update/1 -> Signal Specification/1  "b"
  Signal Specification/1 -> Bus Creator/2
  Signal Specification1/1 -> Bus Creator/1
  connections:
  b/RConn1 -- b Update/RConn1
  W Update/RConn1 -- W/RConn1

== system ad_blocks/forward viewer ==
  Two-Way Connection1 : TwoWayConnection
  Two-Way Connection2 : TwoWayConnection
  X : PMIOPort  Port=1  Side=Left
  Y : PMIOPort  Port=2  Side=Right
  x : Outport
  wires:
  Two-Way Connection1/1 -> Two-Way Connection2/1
  Two-Way Connection2/1 -> x/1, Two-Way Connection1/1
  connections:
  Y/RConn1 -- Two-Way Connection1/RConn1
  X/RConn1 -- Two-Way Connection2/RConn1

== system ad_blocks/inv AD ==
  note: Jx = Jy*(-kron(y',y));
  X : Inport
  JY : Inport  Port=2
  Gain : Gain  Gain=-1
  Product : Product  Inputs=***  Multiplication=Matrix(*)
  Product1 : Product  Inputs=/  Multiplication=Matrix(*)
  Y : Outport
  JX : Outport  Port=2
  wires:
  Product/1 -> JX/1
  X/1 -> Product1/1
  Product1/1 -> Product/3, Gain/1, Y/1
  JY/1 -> Product/2
  Gain/1 -> Product/1

== system ad_blocks/mean all AD ==
  note: All ones scaled by incoming scalar gradient and divided by elements
  Divide : Product  Inputs=*/
  MATLAB System : MATLABSystem  System=MeanGradient_sys  SimulateUsing=Code generation
      mask Type: MeanGradient_sys
      mask Display:
      | disp('MeanGradient_sys');
      | port_label('input',1,'X');
      | port_label('input',2,'JY');
      | port_label('output',1,'JX');
  Sum of Elements : Sum  Inputs=+
  Two-Way Connection : TwoWayConnection
  Two-Way Connection1 : TwoWayConnection
  Width : Width  DataType=single
  X : PMIOPort  Port=1  Side=Left
  Y : PMIOPort  Port=2  Side=Right
  wires:
  Two-Way Connection1/1 -> MATLAB System/1, Width/1, Sum of Elements/1
  Sum of Elements/1 -> Divide/1
  Width/1 -> Divide/2
  MATLAB System/1 -> Two-Way Connection1/1
  Divide/1 -> Two-Way Connection/1
  Two-Way Connection/1 -> MATLAB System/2
  connections:
  Y/RConn1 -- Two-Way Connection/RConn1
  X/RConn1 -- Two-Way Connection1/RConn1

== system ad_blocks/mul AD CC ==
  Two-Way Connection : TwoWayConnection
  Two-Way Connection1 : TwoWayConnection
  Two-Way Connection2 : TwoWayConnection
  mul AD for Scalar FX : ad_blocks/mul AD for Scalar FX
  A : PMIOPort  Port=1  Side=Left
  B : PMIOPort  Port=2  Side=Left
  Y : PMIOPort  Port=3  Side=Right
  wires:
  Two-Way Connection1/1 -> mul AD for Scalar FX/1
  mul AD for Scalar FX/2 -> Two-Way Connection1/1
  Two-Way Connection/1 -> mul AD for Scalar FX/3
  Two-Way Connection2/1 -> mul AD for Scalar FX/2
  mul AD for Scalar FX/3 -> Two-Way Connection2/1
  mul AD for Scalar FX/1 -> Two-Way Connection/1
  connections:
  B/RConn1 -- Two-Way Connection2/RConn1
  A/RConn1 -- Two-Way Connection1/RConn1
  Y/RConn1 -- Two-Way Connection/RConn1

== system ad_blocks/mul AD for Scalar FX ==
  note: J B'
  note: [q,n]
  note: [m,n]
  note: [q,n]
  note: [m,q]
  note: [m,n]
  note: A' J
  note: [m,n]
  note: [m,q]
  note: [q,n]
  note: [m,q]
  A : Inport
  B : Inport  Port=2
  J : Inport  Port=3
  Divide : Product  Inputs=**  Multiplication=Matrix(*)
  MATLAB System : MATLABSystem  System=JBt_sys  SimulateUsing=Code generation
      mask Type: JBt_sys
      mask Display:
      | disp('JBt_sys');
      | port_label('input',1,'J');
      | port_label('input',2,'B');
      | port_label('output',1,'y');
  MATLAB System1 : MATLABSystem  System=AtJ_sys  SimulateUsing=Code generation
      mask Type: AtJ_sys
      mask Display:
      | disp('AtJ_sys');
      | port_label('input',1,'J');
      | port_label('input',2,'A');
      | port_label('output',1,'y');
  Y : Outport
  JA : Outport  Port=2
  JB : Outport  Port=3
  wires:
  Divide/1 -> Y/1
  A/1 -> MATLAB System1/2, Divide/1
  B/1 -> MATLAB System/2, Divide/2
  MATLAB System1/1 -> JB/1
  MATLAB System/1 -> JA/1
  J/1 -> MATLAB System1/1, MATLAB System/1

== system ad_blocks/rehape aD ==
  Two-Way Connection : TwoWayConnection
  Two-Way Connection1 : TwoWayConnection
  function : MATLABSystem  System=ReshapeSystem  shape=shape  SimulateUsing=Interpreted execution
      mask Type: ReshapeSystem
      mask Display:
      | disp('ReshapeSystem');
      | port_label('input',1,'x');
      | port_label('output',1,'y');
  gradient : MATLABSystem  System=ReshapeGradSystem  SimulateUsing=Code generation
      mask Type: ReshapeGradSystem
      mask Display:
      | disp('ReshapeGradSystem');
      | port_label('input',1,'x');
      | port_label('input',2,'J');
      | port_label('output',1,'y');
  X : PMIOPort  Port=1  Side=Left
  Y : PMIOPort  Port=2  Side=Right
  wires:
  function/1 -> Two-Way Connection/1
  Two-Way Connection1/1 -> gradient/1, function/1
  gradient/1 -> Two-Way Connection1/1
  Two-Way Connection/1 -> gradient/2
  connections:
  Y/RConn1 -- Two-Way Connection/RConn1
  X/RConn1 -- Two-Way Connection1/RConn1

== system ad_blocks/softmax_cross_entropy_with_logits ==
  note: logitsmax = max(xlogits,[],classdim); % along class
      | obj.logitsoffsetted = xlogits - repmat(logitsmax,1,classes); % broadcast class
      | scratch = sum(exp(obj.logitsoffsetted),classdim); % exp and sum along class
      | loss = sum((xlabels .* (repmat(log(scratch),1,classes) - obj.logitsoffsetted)),classdim);
      | obj.xvalue = loss;
      | obj.sumx = scratch;
      |
      | classes = size(obj.logits.xvalue,2);
      | J = (exp(obj.logitsoffsetted) ./ repmat(obj.sumx,1,classes))-obj.labels.xvalue;
      | obj.logits.grad(up*J);
  Labels : Inport
  MATLAB System : MATLABSystem  System=softmax_cross_entropy_with_logitsSystem  SimulateUsing=Interpreted execution
      mask Type: softmax_cross_entropy_with_logitsSystem
      mask Display:
      | disp('softmax_cross_entropy_with_logitsSystem');
      | port_label('input',1,'xlogits');
      | port_label('input',2,'xlabels');
      | port_label('output',1,'loss');
      | port_label('output',2,'logitsoffsetted');
      | port_label('output',3,'sumx');
  MATLAB System1 : MATLABSystem  System=softmax_cross_entropy_with_logitsGradSystem  SimulateUsing=Code generation
      mask Type: softmax_cross_entropy_with_logitsGradSystem
      mask Display:
      | disp('softmax_cross_entropy_with_logitsGradSystem');
      | port_label('input',1,'logits');
      | port_label('input',2,'labels');
      | port_label('input',3,'Jin');
      | port_label('input',4,'logitsoffsetted');
      | port_label('input',5,'sumx');
      | port_label('output',1,'J');
  Two-Way Connection : TwoWayConnection
  Two-Way Connection1 : TwoWayConnection
  function : MATLAB Function  Commented=on  TreatAsAtomicUnit=on
  gradient : MATLAB Function  Commented=on  TreatAsAtomicUnit=on
  Logits : PMIOPort  Port=1  Side=Left
  Y : PMIOPort  Port=2  Side=Right
  wires:
  Two-Way Connection1/1 -> MATLAB System1/1, MATLAB System/1
  MATLAB System1/1 -> Two-Way Connection1/1
  Two-Way Connection/1 -> MATLAB System1/3
  Labels/1 -> MATLAB System1/2, MATLAB System/2
  MATLAB System/1 -> Two-Way Connection/1
  MATLAB System/2 -> MATLAB System1/4
  MATLAB System/3 -> MATLAB System1/5
  connections:
  Logits/RConn1 -- Two-Way Connection1/RConn1
  Y/RConn1 -- Two-Way Connection/RConn1

== system ad_blocks/transpose vector AD ==
  note: The incoming JX is [p,q, m, 1] and the output [p,q,1,m]
      | The compact form becomes [pq,m] as [pq,m] so no changes
  X : Inport
  JY : Inport  Port=2
  Permute Dimensions : PermuteDimensions
  Y : Outport
  JX : Outport  Port=2
  wires:
  JY/1 -> JX/1
  Permute Dimensions/1 -> Y/1
  X/1 -> Permute Dimensions/1

== system ad_blocks/Adam Old/Moment Update ==
  beta : Inport
  X for 1-beta : Inport  Port=2
  X for beta : Inport  Port=3
  Add : Sum  InputSameDT=on  OutDataTypeStr=Inherit: Same as first input
  MATLAB Function : MATLAB Function  TreatAsAtomicUnit=on
  Product1 : Product
  Product2 : Product
  Y : Outport
  wires:
  Add/1 -> Y/1
  Product1/1 -> Add/1
  MATLAB Function/1(y) -> Product1/1
  X for beta/1 -> Product2/2
  X for 1-beta/1 -> Product1/2
  beta/1 -> MATLAB Function/1(u), Product2/1
  Product2/1 -> Add/2

== system ad_blocks/Adam Old/Second Moment Update ==
  beta : Inport
  X for 1-beta : Inport  Port=2
  X for beta : Inport  Port=3
  Add : Sum
  MATLAB Function : MATLAB Function  TreatAsAtomicUnit=on
  Product1 : Product
  Product2 : Product
  Y : Outport
  wires:
  Product2/1 -> Add/2
  beta/1 -> Product2/1, MATLAB Function/1(u)
  X for 1-beta/1 -> Product1/2
  X for beta/1 -> Product2/2
  MATLAB Function/1(y) -> Product1/1
  Product1/1 -> Add/1
  Add/1 -> Y/1

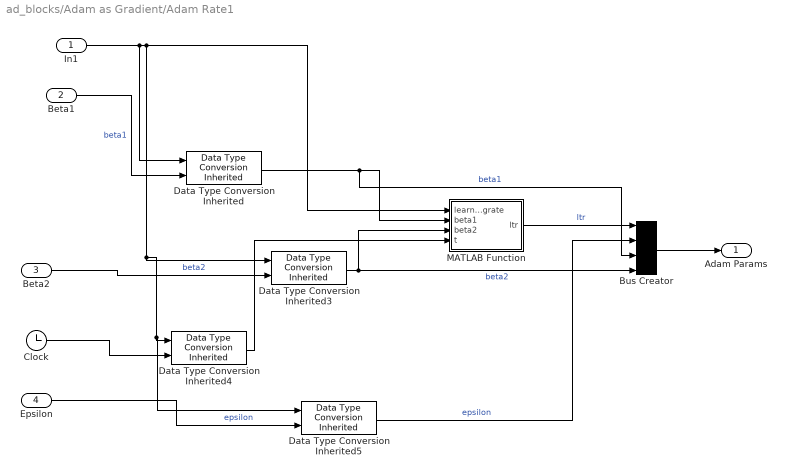
== system ad_blocks/Adam as Gradient/Adam Rate1 ==
  In1 : Inport
  Beta1 : Inport  Port=2
  Beta2 : Inport  Port=3
  Epsilon : Inport  Port=4
  Bus Creator : BusCreator  Inputs=4
  Clock : Clock
  Data Type Conversion Inherited{,3..5} (4 alike) : simulink/Signal Attributes/Data Type Conversion Inherited  ConvertRealWorld=Real World Value  DoSatur=off
      settings: SourceProductName=Simulink  SourceProductBaseCode=SL
  MATLAB Function : MATLAB Function  TreatAsAtomicUnit=on
  Adam Params : Outport
  wires:
  MATLAB Function/1(ltr) -> Bus Creator/1  "ltr"
  Bus Creator/1 -> Adam Params/1
  Data Type Conversion Inherited/1 -> Bus Creator/3, MATLAB Function/2(beta1)  "beta1"
  In1/1 -> Data Type Conversion Inherited/1, Data Type Conversion Inherited5/1, Data Type Conversion Inherited4/1, Data Type Conversion Inherited3/1, MATLAB Function/1(learningrate)
  Beta1/1 -> Data Type Conversion Inherited/2  "beta1"
  Beta2/1 -> Data Type Conversion Inherited3/2  "beta2"
  Data Type Conversion Inherited3/1 -> MATLAB Function/3(beta2), Bus Creator/4  "beta2"
  Clock/1 -> Data Type Conversion Inherited4/2
  Data Type Conversion Inherited4/1 -> MATLAB Function/4(t)
  Epsilon/1 -> Data Type Conversion Inherited5/2  "epsilon"
  Data Type Conversion Inherited5/1 -> Bus Creator/2  "epsilon"

== system ad_blocks/Dropout 23/If full ==
  x : Inport
  J : Inport  Port=2
  Action Port : ActionPort
  y : Outport
  Jx : Outport  Port=2
  wires:
  x/1 -> y/1
  J/1 -> Jx/1

== system ad_blocks/Dropout 23/If rate ==
  x : Inport
  J : Inport  Port=2
  rate : Inport  Port=3
  Action Port : ActionPort
  MATLAB System : MATLABSystem  System=dropout_sys  SimulateUsing=Code generation
      mask Type: dropout_sys
      mask Display:
      | disp('dropout_sys');
      | port_label('input',1,'x');
      | port_label('input',2,'rate');
      | port_label('output',1,'y');
      | port_label('output',2,'mask');
  Product : Product
  y : Outport
  Jx : Outport  Port=2
  wires:
  x/1 -> MATLAB System/1
  rate/1 -> MATLAB System/2
  MATLAB System/1 -> y/1
  MATLAB System/2 -> Product/2
  J/1 -> Product/1
  Product/1 -> Jx/1

== system ad_blocks/MNIST Train Test/Case Test ==
  Action Port : ActionPort
  Test  Set1 : Subsystem  mask{IsTrainSet=off, BatchSize=BatchSize}
  Y : Outport
  Yhot : Outport  Port=2
  X : Outport  Port=3
  indices : Outport  Port=4
  wires:
  Test  Set1/1(Y) -> Y/1
  Test  Set1/2(Yhot) -> Yhot/1
  Test  Set1/3(X) -> X/1
  Test  Set1/4(indices) -> indices/1

== system ad_blocks/MNIST Train Test/Case Train ==
  Action Port : ActionPort
  Train Set : Subsystem  mask{IsTrainSet=on, BatchSize=BatchSize}
  Y : Outport
  Yhot : Outport  Port=2
  X : Outport  Port=3
  indices : Outport  Port=4
  wires:
  Train Set/1(Y) -> Y/1
  Train Set/2(Yhot) -> Yhot/1
  Train Set/3(X) -> X/1
  Train Set/4(indices) -> indices/1

== system ad_blocks/MNIST Train Test/Case Test/Test  Set1 ==
  MATLAB System : MATLABSystem  System=MnistSystemInt  trainset=IsTrainSet  items=BatchSize  shuffle=0  SimulateUsing=Interpreted execution
      mask Type: MnistSystemInt
      mask Display:
      | disp('MnistSystemInt');
      | port_label('output',1,'indices');
  S-Function1 : S-Function  FunctionName=sfun_loadmnist  Parameters=IsTrainSet  SFunctionDeploymentMode=off  EnableBusSupport=off
  Terminator2 : Terminator
  Variable Selector : dspindex/Variable Selector  NumInputs=3  rowsOrCols=Rows  IdxMode=Variable  Elements=[1 3]  ZerOneIdxMode=One-based  errmode=Generate Error  FillMode=on  FillValues=0
  Y : Outport
  Yhot : Outport  Port=2
  X : Outport  Port=3
  indices : Outport  Port=4
  wires:
  S-Function1/2 -> Variable Selector/2
  Variable Selector/2 -> Y/1
  Variable Selector/1 -> X/1
  MATLAB System/1 -> indices/1, Variable Selector/4
  Variable Selector/3 -> Yhot/1
  S-Function1/3 -> Variable Selector/3
  S-Function1/4 -> Variable Selector/1
  S-Function1/1 -> Terminator2/1

== system ad_blocks/MNIST Train Test/Case Train/Train Set ==
  MATLAB System : MATLABSystem  System=MnistSystemInt  trainset=IsTrainSet  items=BatchSize  shuffle=0  SimulateUsing=Interpreted execution
      mask Type: MnistSystemInt
      mask Display:
      | disp('MnistSystemInt');
      | port_label('output',1,'indices');
  S-Function1 : S-Function  FunctionName=sfun_loadmnist  Parameters=IsTrainSet  SFunctionDeploymentMode=off  EnableBusSupport=off
  Terminator2 : Terminator
  Variable Selector : dspindex/Variable Selector  NumInputs=3  rowsOrCols=Rows  IdxMode=Variable  Elements=[1 3]  ZerOneIdxMode=One-based  errmode=Generate Error  FillMode=on  FillValues=0
  Y : Outport
  Yhot : Outport  Port=2
  X : Outport  Port=3
  indices : Outport  Port=4
  wires:
  S-Function1/1 -> Terminator2/1
  S-Function1/4 -> Variable Selector/1
  S-Function1/3 -> Variable Selector/3
  Variable Selector/3 -> Yhot/1
  MATLAB System/1 -> indices/1, Variable Selector/4
  Variable Selector/1 -> X/1
  Variable Selector/2 -> Y/1
  S-Function1/2 -> Variable Selector/2

== matlab function ad_blocks/Adam Descent Masked/MATLAB Function ==
  data: learningrate input; ltr output; beta1 input; beta2 input; t input
function ltr = fcn(learningrate,beta1,beta2,t)

if beta1 == 1 || beta2 == 1
    ltr = -learningrate;
else
    ltr = - learningrate * sqrt(1 - beta2^t) / (1 - beta1^t);
end

== matlab function ad_blocks/Adam Rate/MATLAB Function ==
  data: learningrate input; ltr output; beta1 input; beta2 input; t input
function ltr = fcn(learningrate,beta1,beta2,t)

if beta1 == 1 || beta2 == 1
    ltr = -learningrate;
else
    ltr = - learningrate * sqrt(1 - beta2^t) / (1 - beta1^t);
end
